simulink model "Controllo_Simulazione"  (R2020b)
settings: Solver=FixedStepDiscrete  StartTime=0.0  StopTime=5  FixedStep=0.001  RelTol=1e-3
undefined symbols (not defined in the file or in its folder): DiscIntNeverNeededParam
libraries: simulink x7, simulink_extras x2
settings Model: Creator=daniele_ravasio  LastModifiedBy=simoc

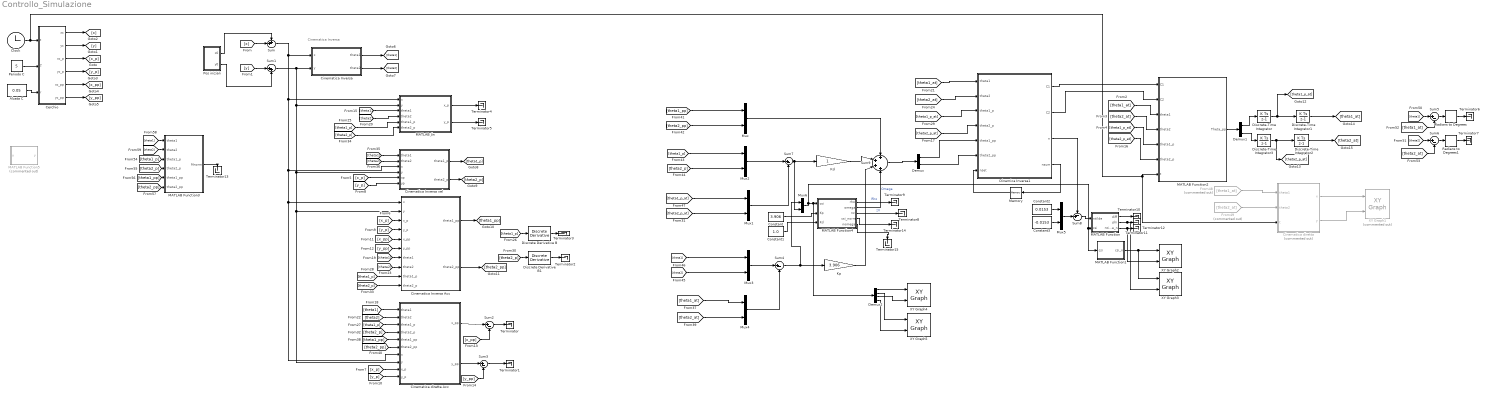
== system Controllo_Simulazione ==
  note: Cinematica Inversa
  Alzata C : Constant  Value=0.05
  Cerchio : MATLAB Function  TreatAsAtomicUnit=on
  Cinematica Inversa : MATLAB Function  TreatAsAtomicUnit=on
  Cinematica Inversa Acc : MATLAB Function  TreatAsAtomicUnit=on
  Cinematica Inversa vel : MATLAB Function  TreatAsAtomicUnit=on
  Cinematica diretta : MATLAB Function  Commented=on  TreatAsAtomicUnit=on
  Cinematica diretta Acc : MATLAB Function  TreatAsAtomicUnit=on
  Clock : Clock
  Constant : Constant  Value=3.906
  Constant1 : Constant  Value=1.0
  Constant2 : Constant  Value=0.0153
  Constant3 : Constant  Value=-0.0153
  Demux : Demux  Outputs=2
  Demux1 : Demux  Outputs=2
  Demux2 : Demux
  Dinamica Inversa1 : MATLAB Function  TreatAsAtomicUnit=on
  Discrete Derivative B : simulink/Discrete/Discrete Derivative  gainval=1.0  ICPrevScaledInput=0.0  OutMin=[]  OutMax=[]  OutDataType=fixdt(1, 16)  OutScaling=2^-10  DoSatur=off
  Discrete Derivative B1 : simulink/Discrete/Discrete Derivative  gainval=1.0  ICPrevScaledInput=0.0  OutMin=[]  OutMax=[]  OutDataType=fixdt(1, 16)  OutScaling=2^-10  DoSatur=off
  Discrete-Time Integrator : DiscreteIntegrator  SampleTime=-1  ICPrevOutput=DiscIntNeverNeededParam  ICPrevScaledInput=DiscIntNeverNeededParam
  Discrete-Time Integrator1 : DiscreteIntegrator  InitialCondition=deg2rad(100)  SampleTime=-1  ICPrevOutput=DiscIntNeverNeededParam  ICPrevScaledInput=DiscIntNeverNeededParam
  Discrete-Time Integrator2 : DiscreteIntegrator  InitialCondition=deg2rad(80)  SampleTime=-1  ICPrevOutput=DiscIntNeverNeededParam  ICPrevScaledInput=DiscIntNeverNeededParam
  Discrete-Time Integrator3 : DiscreteIntegrator  SampleTime=-1  ICPrevOutput=DiscIntNeverNeededParam  ICPrevScaledInput=DiscIntNeverNeededParam
  From48 : From  Commented=on  GotoTag=theta1_at
  From49 : From  Commented=on  GotoTag=theta2_at
  Kd : Gain
  Kp : Gain  Gain=3.906
  MATLAB Function : MATLAB Function  TreatAsAtomicUnit=on
  MATLAB Function1 : MATLAB Function  TreatAsAtomicUnit=on
  MATLAB Function2 : MATLAB Function  TreatAsAtomicUnit=on
  MATLAB Function3 : MATLAB Function  TreatAsAtomicUnit=on
  MATLAB Function4 : MATLAB Function  TreatAsAtomicUnit=on
  MATLAB Function5 : MATLAB Function  Commented=on  TreatAsAtomicUnit=on
  MATLAB Jin : MATLAB Function  TreatAsAtomicUnit=on
  Memory : Memory
  Mux{,1..6} (7 alike) : Mux  Inputs=2
  Periodo C : Constant  Value=5
  Pos iniziali : Subsystem
  Radians to Degrees : simulink_extras/Transformations/Radians to Degrees
  Radians to Degrees1 : simulink_extras/Transformations/Radians to Degrees
  Sum : Sum  Inputs=++|
  Sum1 : Sum  Inputs=|++
  Sum{2..7} (6 alike) : Sum  Inputs=|+-
  Sum8 : Sum  Inputs=-+|
  Sum9 : Sum  Inputs=+|+|+|+
  Terminator{,1..15} (16 alike) : Terminator
  XY Graph1 : simulink/Sinks/XY Graph  Commented=on  xmin=-0.15  xmax=0.15  ymin=0  ymax=0.5  st=0.001
  XY Graph2 : simulink/Sinks/XY Graph  xmin=0  xmax=0.01  ymin=0  ymax=0.05  st=0.001
  XY Graph3 : simulink/Sinks/XY Graph  xmin=0  xmax=0.01  ymin=0  ymax=0.1  st=0.001
  XY Graph4 : simulink/Sinks/XY Graph  xmin=0  xmax=0.01  ymin=0  ymax=0.1  st=0.001
  XY Graph5 : simulink/Sinks/XY Graph  xmin=0  xmax=0.01  ymin=0  ymax=0.1  st=0.001
  wires:
  Clock/1 -> MATLAB Function2/7(t), Cinematica diretta/3(t), Cerchio/1(t)
  Alzata C/1 -> Cerchio/3(r)
  Periodo C/1 -> Cerchio/2(T)
  Mux1/1 -> Sum7/2
  [x_pp] -> Sum2/2
  Cerchio/5(xc_pp) -> [x_pp]
  Pos iniziali/1(x0) -> Sum/1
  [theta1] -> Cinematica Inversa Acc/7(theta1)
  Demux/2 -> Dinamica Inversa1/6(theta2_pp)
  [theta1] -> Cinematica Inversa vel/1(theta1)
  [theta1_p] -> Discrete Derivative B/1
  [x_p] -> Cinematica Inversa vel/5(xp)
  Cinematica diretta Acc/2(y_pp) -> Sum3/1
  Cerchio/1(xc) -> [x]
  Cerchio/3(xc_p) -> [x_p]
  [theta2] -> Cinematica Inversa Acc/8(theta2)
  [theta1] -> Cinematica diretta Acc/1(theta1)
  Cinematica Inversa Acc/1(theta1_pp) -> [theta1_pp]
  Kd/1 -> Sum9/2
  Mux/1 -> Sum9/1
  Cinematica Inversa/1(theta1) -> [theta1]
  [theta2_p] -> MATLAB Jin/6(theta2_p)
  Cinematica diretta/2(y) -> XY Graph1/2
  [x_p] -> Cinematica diretta Acc/9(x_p)
  Cinematica diretta/1(x) -> XY Graph1/1
  Kp/1 -> Sum9/3
  Demux/1 -> Dinamica Inversa1/5(theta1_pp)
  Mux3/1 -> Sum4/1
  Cinematica Inversa vel/2(theta2_p) -> [theta2_p]
  Sum4/1 -> Mux6/1, Kp/1
  Mux4/1 -> Sum4/2
  [theta2] -> Cinematica Inversa vel/2(theta2)
  [theta1_p] -> Cinematica diretta Acc/3(theta1_p)
  [theta2_p] -> Cinematica diretta Acc/4(theta2_p)
  Sum3/1 -> Terminator1/1
  Mux2/1 -> Sum7/1
  MATLAB Jin/1(x_p) -> Terminator4/1
  [x] -> Sum/2
  Sum7/1 -> Mux6/2, Kd/1
  Sum9/1 -> Demux/1
  [y_pp] -> Cinematica Inversa Acc/6(y_pp)
  Pos iniziali/2(y0) -> Sum1/2
  [theta1_p] -> MATLAB Jin/5(theta1_p)
  [theta1_pp] -> Cinematica diretta Acc/5(theta1_pp)
  [y] -> Sum1/1
  Cinematica Inversa vel/1(theta1_p) -> [theta1_p]
  [y_p] -> Cinematica Inversa vel/6(yp)
  [y_pp] -> Sum3/2
  [theta1] -> MATLAB Jin/3(theta1)
  [y_p] -> Cinematica Inversa Acc/4(y_p)
  Cinematica Inversa/2(theta2) -> [theta2]
  Sum2/1 -> Terminator/1
  [theta2] -> MATLAB Jin/4(theta2)
  [x_p] -> Cinematica Inversa Acc/3(x_p)
  [y_p] -> Cinematica diretta Acc/10(y_p)
  [x_pp] -> Cinematica Inversa Acc/5(x_pp)
  [theta2] -> Cinematica diretta Acc/2(theta2)
  MATLAB Jin/2(y_p) -> Terminator5/1
  [theta2_p] -> Cinematica Inversa Acc/10(theta2_p)
  Cinematica diretta Acc/1(x_pp) -> Sum2/1
  [theta2_p] -> Discrete Derivative B1/1
  Cerchio/4(yc_p) -> [y_p]
  Cerchio/6(yc_pp) -> [y_pp]
  [theta1_p] -> Cinematica Inversa Acc/9(theta1_p)
  [theta2_pp] -> Cinematica diretta Acc/6(theta2_pp)
  Cerchio/2(yc) -> [y]
  Sum1/1 -> Cinematica Inversa Acc/2(y), Cinematica diretta Acc/8(y), Cinematica Inversa vel/4(y), MATLAB Jin/2(y), Cinematica Inversa/2(y)
  Sum/1 -> Cinematica Inversa Acc/1(x), Cinematica diretta Acc/7(x), Cinematica Inversa vel/3(x), MATLAB Jin/1(x), Cinematica Inversa/1(x)
  [theta1_pp] -> Mux/1
  [theta2_pp] -> Mux/2
  [theta2_p] -> Mux2/2
  [theta1_p] -> Mux2/1
  Dinamica Inversa1/1(C1) -> MATLAB Function2/1(C1)
  Dinamica Inversa1/2(C2) -> MATLAB Function2/2(C2)
  MATLAB Function2/1(Theta_pp) -> Demux1/1
  Demux1/1 -> Discrete-Time Integrator/1
  Demux1/2 -> Discrete-Time Integrator3/1
  Discrete-Time Integrator3/1 -> Discrete-Time Integrator2/1, [theta2_p_at]
  Discrete-Time Integrator/1 -> Discrete-Time Integrator1/1, [theta1_p_at]
  [theta1_at] -> MATLAB Function2/3(theta1)
  [theta2_at] -> MATLAB Function2/4(theta2)
  Discrete-Time Integrator1/1 -> [theta1_at]
  Discrete-Time Integrator2/1 -> [theta2_at]
  [theta1_p_at] -> MATLAB Function2/5(theta1_p)
  [theta2_p_at] -> MATLAB Function2/6(theta2_p)
  [theta1_p_at] -> Dinamica Inversa1/3(theta1_p)
  [theta2_p_at] -> Dinamica Inversa1/4(theta2_p)
  [theta1_at] -> Mux4/1
  [theta2_at] -> Mux4/2
  From49/1 -> Cinematica diretta/2(theta2)
  From48/1 -> Cinematica diretta/1(theta1)
  [theta1_p_at] -> Mux1/1
  [theta2_p_at] -> Mux1/2
  [theta1] -> Mux3/1
  [theta2] -> Mux3/2
  [theta1_at] -> Dinamica Inversa1/1(theta1)
  [theta2_at] -> Dinamica Inversa1/2(theta2)
  [theta1] -> Sum5/1
  [theta1_at] -> Sum5/2
  [theta2] -> Sum6/1
  [theta2_at] -> Sum6/2
  Sum5/1 -> Radians to Degrees/1
  Radians to Degrees/1 -> Terminator6/1
  Sum6/1 -> Radians to Degrees1/1
  Radians to Degrees1/1 -> Terminator7/1
  Cinematica Inversa Acc/2(theta2_pp) -> [theta2_pp]
  Discrete Derivative B1/1 -> Terminator2/1
  Discrete Derivative B/1 -> Terminator3/1
  MATLAB Function4/2(omega) -> Sum9/4  "Omega"
  Constant/1 -> MATLAB Function4/2(Kp)
  Constant1/1 -> MATLAB Function4/3(Kd)
  MATLAB Function4/1(rho) -> Terminator9/1  "Rho"
  Dinamica Inversa1/4(nsum) -> Memory/1
  Memory/1 -> Dinamica Inversa1/7(nset)
  Dinamica Inversa1/3(n) -> Sum8/1
  Constant2/1 -> Mux5/1
  Constant3/1 -> Mux5/2
  Mux5/1 -> Sum8/2
  Sum8/1 -> MATLAB Function/1(ntilde)
  Mux6/1 -> Demux2/1, MATLAB Function4/1(csi), MATLAB Function1/1(csi), MATLAB Function/2(csi)
  MATLAB Function/1(diff) -> Terminator10/1
  MATLAB Function/2(phi) -> XY Graph3/2, Terminator11/1
  MATLAB Function1/1(csi_n) -> XY Graph3/1, XY Graph2/1
  MATLAB Function/3(ntilde_n) -> XY Graph2/2, Terminator12/1
  [theta1_p] -> MATLAB Function3/3(theta1_p)
  [theta2_p] -> MATLAB Function3/4(theta2_p)
  [theta1_pp] -> MATLAB Function3/5(theta1_pp)
  [theta2_pp] -> MATLAB Function3/6(theta2_pp)
  [theta1] -> MATLAB Function3/1(theta1)
  [theta2] -> MATLAB Function3/2(theta2)
  MATLAB Function3/1(Mnorm) -> Terminator13/1
  MATLAB Function4/4(csi_norm) -> Terminator14/1
  MATLAB Function4/5(nomega) -> Terminator15/1
  MATLAB Function4/3(nz) -> Terminator8/1  "zV"
  Demux2/1 -> XY Graph4/1
  Demux2/3 -> XY Graph4/2
  Demux2/2 -> XY Graph5/1
  Demux2/4 -> XY Graph5/2

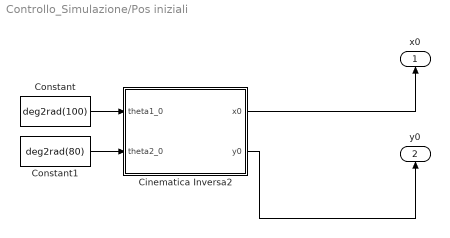
== system Controllo_Simulazione/Pos iniziali ==
  Cinematica Inversa2 : MATLAB Function  TreatAsAtomicUnit=on
  Constant : Constant  Value=deg2rad(100)
  Constant1 : Constant  Value=deg2rad(80)
  x0 : Outport
  y0 : Outport  Port=2
  wires:
  Cinematica Inversa2/1(x0) -> x0/1
  Cinematica Inversa2/2(y0) -> y0/1
  Constant/1 -> Cinematica Inversa2/1(theta1_0)
  Constant1/1 -> Cinematica Inversa2/2(theta2_0)

== matlab function Controllo_Simulazione/Cinematica diretta ==
  data: x output; theta1 input; y output; theta2 input; t input
function [x, y] = fcn(theta1, theta2,t)
d = 0.09;
l = 0.25;


A = l^2*(sin(theta2)-sin(theta1))^2 + (-2*d -l*(cos(theta2)-cos(theta1)))^2;
B = -2*l^2*d*(sin(theta2)-sin(theta1))*(cos(theta2)+cos(theta1)) + ...
    l*(sin(theta2)-sin(theta1))*(-2*d -l*(cos(theta2)-cos(theta1)))*(-2*d -2*l*cos(theta2)) - ...
    2*l*sin(theta2)*(-2*d -l*(cos(theta2)-cos(theta1)))^2;
C = l^2*d^2*(cos(theta2)+cos(theta1))^2 -l*d*(cos(theta2)+cos(theta1))*(-2*d -l*(cos(theta2)-cos(theta1)))*(-2*d -2*l*cos(theta2)) + ...
    (d^2 + 2*d*l*cos(theta2))*(-2*d - l*(cos(theta2)-cos(theta1)))^2;

% Posizione Y end-effector
y =  (-B + sqrt(B^2 - 4*A*C))/(2*A);
% Posizione X end-effector
x =  (y*l*(sin(theta2)-sin(theta1)) - l*d*(cos(theta2)+cos(theta1)))/(-2*d -l*(cos(theta2)-cos(theta1)));
end

== matlab function Controllo_Simulazione/Pos iniziali/Cinematica Inversa2 ==
  data: theta1_0 input; theta2_0 input; x0 output; y0 output
function [x0, y0] = fcn(theta1_0, theta2_0)

d = 0.09; 
l = 0.25;

A = l^2*(sin(theta2_0)-sin(theta1_0))^2 + (-2*d -l*(cos(theta2_0)-cos(theta1_0)))^2;
B = -2*l^2*d*(sin(theta2_0)-sin(theta1_0))*(cos(theta2_0)+cos(theta1_0)) + ...
    l*(sin(theta2_0)-sin(theta1_0))*(-2*d -l*(cos(theta2_0)-cos(theta1_0)))*(-2*d -2*l*cos(theta2_0)) - ...
    2*l*sin(theta2_0)*(-2*d -l*(cos(theta2_0)-cos(theta1_0)))^2;
C = l^2*d^2*(cos(theta2_0)+cos(theta1_0))^2 -l*d*(cos(theta2_0)+cos(theta1_0))*(-2*d -l*(cos(theta2_0)-cos(theta1_0)))*(-2*d -2*l*cos(theta2_0)) + ...
    (d^2 + 2*d*l*cos(theta2_0))*(-2*d - l*(cos(theta2_0)-cos(theta1_0)))^2;

% Posizione Y end-effector
y0 = (-B + sqrt(B^2 - 4*A*C))/(2*A);
% Posizione X end-effector
x0 = (y0*l*(sin(theta2_0)-sin(theta1_0)) - l*d*(cos(theta2_0)+cos(theta1_0)))/(-2*d -l*(cos(theta2_0)-cos(theta1_0)));

== matlab function Controllo_Simulazione/Cinematica Inversa ==
  data: x input; theta1 output; y input; theta2 output
function [theta1, theta2] = fcn(x, y)

d = 0.09; 
l = 0.25;

p = 2*d*l + 2*x*l;
e = 2*y*l;
f = x^2 + d^2 + y^2 + 2*x*d;
a = -2*d*l + 2*x*l;
b = +2*y*l;
c = x^2 + d^2 + y^2 - 2*x*d;



   theta1 = 2*atan2(e + sqrt(p^2 + e^2 -f^2), p +f);


   theta2 = 2*atan2(b - sqrt(a^2 + b^2 -c^2), a +c);
   if (theta2) < -deg2rad(200)
       theta2 = theta2 + 2*pi;
   end

== matlab function Controllo_Simulazione/Cinematica Inversa vel ==
  data: theta1 input; theta2 input; x input; y input; xp input; theta1_p output; yp input; theta2_p output
function [theta1_p, theta2_p] = fcn(theta1, theta2,x, y, xp, yp)

d = 0.09; 
l = 0.25;

N21 = -l*sin(theta1)*(x+d-l*cos(theta1)) + l*cos(theta1)*(y-l*sin(theta1));

N22 = -l*cos(theta2)*(y-l*sin(theta2))*(x+d-l*cos(theta1))/(x-d-l*cos(theta2)) + l*sin(theta2)*(x+d-l*cos(theta1));

D2 = y-l*sin(theta1) - (y-l*sin(theta2))*(x+d-l*cos(theta1))/(x-d-l*cos(theta2));

J21 = N21/D2;

J22 = N22/D2;

J11 = -(y-l*sin(theta2))/(x-d-l*cos(theta2))*(J21);

J12 = -(y-l*sin(theta2))/(x-d-l*cos(theta2))*(J22) -l*sin(theta2) + (y-l*sin(theta2))/(x-d-l*cos(theta2))*(l*cos(theta2));

J = [J11 J12; J21 J22];

theta_p = J^-1 * [xp; yp];
theta1_p = theta_p(1);
theta2_p = theta_p(2);

== matlab function Controllo_Simulazione/MATLAB Jin ==
  data: x input; y input; theta1 input; x_p output; theta2 input; theta1_p input; theta2_p input; y_p output
function [x_p, y_p] = fcn(x, y, theta1, theta2, theta1_p, theta2_p)

d = 0.09; 
l = 0.25;

N21 = -l*sin(theta1)*(x+d-l*cos(theta1)) + l*cos(theta1)*(y-l*sin(theta1));

N22 = -l*cos(theta2)*(y-l*sin(theta2))*(x+d-l*cos(theta1))/(x-d-l*cos(theta2)) + l*sin(theta2)*(x+d-l*cos(theta1));

D2 = y-l*sin(theta1) - (y-l*sin(theta2))*(x+d-l*cos(theta1))/(x-d-l*cos(theta2));

J21 = N21/D2;

J22 = N22/D2;

J11 = -(y-l*sin(theta2))/(x-d-l*cos(theta2))*(J21);

J12 = -(y-l*sin(theta2))/(x-d-l*cos(theta2))*(J22) -l*sin(theta2) + (y-l*sin(theta2))/(x-d-l*cos(theta2))*(l*cos(theta2));

x_p = J11*theta1_p + J12*theta2_p;
y_p = J21*theta1_p + J22*theta2_p;

== matlab function Controllo_Simulazione/Cerchio ==
  data: xc output; t input; yc output; T input; r input; xc_p output; yc_p output; xc_pp output; yc_pp output
function [xc, yc, xc_p, yc_p, xc_pp, yc_pp] = fcn(t, T, r)
xv = 0.4;
xj = 0.1;
x = t/T;
Ca = 1/((1-xv)*(xv-xj));
if ( x >= 0 && x < xj)            %acc crescente positiva
    f = Ca/xj*x;
    F = (1/2)*Ca/xj*x^2;
    G = (1/6)*Ca/xj*x^3;
    J = Ca/xj;

  elseif (x >= xj && x < (xv-xj))   %acc costante positiva
    f = Ca;
    F = Ca*x - (1/2)*Ca*xj;
    G = (1/2)*Ca*x^2 - (1/2)*Ca*xj*x + (1/6)*Ca*xj^2;
    J = 0;

  elseif( x>= (xv-xj) && x < xv)    %acc decrescente positiva
    f = -Ca/xj*x + Ca*xv/xj;
    F = -(1/2)*Ca/xj*x^2 + Ca/xj*xv*x - Ca*(xj + (1/2)/xj*xv^2 - xv);
    G = -(1/6)*Ca/xj*x^3 + (1/2)*Ca/xj*xv*x^2 - Ca*(xj + (1/2)/xj*xv^2 - xv)*x ...
        - (1/2)*Ca*xv^2  + (1/6)*Ca/xj*xv^3 + (1/2)*Ca*xv*xj;
    J = -Ca/xj;

  elseif( x>= xv && x < (1-xv))     %acc costante nulla
    f = 0;
    F = Ca*(xv - xj);
    G = Ca*(xv - xj)*x - (1/2)*Ca*xv^2 + (1/2)*Ca*xv*xj;
    J = 0;
    
  elseif( x>= (1-xv) && x < (1-xv+xj))   %acc decrescente negativa
    f = -Ca/xj*x + Ca/xj*(1-xv);
    F = -(1/2)*Ca/xj*x^2 + Ca/xj*(1-xv)*x + Ca*(xv-xj) - (1/2)*Ca/xj*(1-xv)^2;
    G = -(1/6)*Ca/xj*x^3 + (1/2)*Ca/xj*(1-xv)*x^2 + Ca*(xv-xj)*x - (1/2)*Ca/xj*(1-xv)^2*x ...
        - (1/2)*Ca*xv^2 + (1/2)*Ca*xv*xj + (1/6)*Ca/xj*(1-xv)^3;
    J = -Ca/xj;
    
  elseif( x>= (1-xv+xj) && x < (1-xj))   %acc costante negativa
    f = -Ca; 
    F = -Ca*x + Ca - (1/2)*Ca*xj;
    G = -(1/2)*Ca*x^2 + Ca*x - (1/2)*Ca*xj*x + 1 - Ca*(-(1/2)*xj + (1/6)*xj^2 + (1/2));
    J = 0;
    
  elseif( x>= (1-xj) && x <= 1)          %acc crescente negativa
    f = Ca/xj*(x-1);
    F = (1/2)*Ca/xj*x^2 - Ca/xj*x +(1/2)*Ca/xj;
    G = (1/6)*Ca/xj*x^3 - (1/2)*Ca/xj*x^2 +(1/2)*Ca/xj*x + 1 - (1/6)*Ca/xj;
    J = Ca/xj;
    
  else                                   %acc costante nulla
    f = 0;
    F = 0;
    G = 1;
    J = 0;
end
  
 alfa = G*2*pi;
 alfa_p = F*2*pi/T;
 alfa_pp = f*2*pi/(T^2);
 xc = r*cos(pi/2-alfa);
 yc = r*sin(pi/2-alfa) - r;
 xc_p = r*sin(pi/2-alfa)*alfa_p;
 yc_p = -r*cos(pi/2-alfa)*alfa_p;
 xc_pp = -r*cos(pi/2-alfa)*alfa_p^2 + r*sin(pi/2-alfa)*alfa_pp;
 yc_pp = -r*sin(pi/2-alfa)*alfa_p^2- r*cos(pi/2-alfa)*alfa_pp;

== matlab function Controllo_Simulazione/Cinematica Inversa Acc ==
  data: x input; y input; x_p input; y_p input; x_pp input; y_pp input; theta1 input; theta2 input; theta1_pp output; theta1_p input; theta2_p input; theta2_pp output
function [theta1_pp, theta2_pp] = CinInvAcc(x, y, x_p, y_p, x_pp, y_pp, theta1, theta2, theta1_p,theta2_p)

d = 0.09; 
l = 0.25;

N21 = -l*sin(theta1)*(x+d-l*cos(theta1)) + l*cos(theta1)*(y-l*sin(theta1));

N22 = -l*cos(theta2)*(y-l*sin(theta2))*(x+d-l*cos(theta1))/(x-d-l*cos(theta2)) + l*sin(theta2)*(x+d-l*cos(theta1));

D2 = y-l*sin(theta1) - (y-l*sin(theta2))*(x+d-l*cos(theta1))/(x-d-l*cos(theta2));

J21 = N21/D2;

J22 = N22/D2;

J11 = -(y-l*sin(theta2))/(x-d-l*cos(theta2))*(J21);

J12 = -(y-l*sin(theta2))/(x-d-l*cos(theta2))*(J22) -l*sin(theta2) + (y-l*sin(theta2))/(x-d-l*cos(theta2))*(l*cos(theta2));

J = [J11 J12; J21 J22];

J_p11 = ((l*cos(theta1)*(y - l*sin(theta1)) - l*sin(theta1)*(d + x - l*cos(theta1)))*(y_p - l*cos(theta2)*theta2_p))/((d - x + l*cos(theta2))*(y - l*sin(theta1) + ((y - l*sin(theta2))*(d + x - l*cos(theta1)))/(d - x + l*cos(theta2)))) - ((y - l*sin(theta2))*(l*sin(theta1)*(x_p + l*sin(theta1)*theta1_p) - l*cos(theta1)*(y_p - l*cos(theta1)*theta1_p) + l*sin(theta1)*(y - l*sin(theta1))*theta1_p + l*cos(theta1)*theta1_p*(d + x - l*cos(theta1))))/((d - x + l*cos(theta2))*(y - l*sin(theta1) + ((y - l*sin(theta2))*(d + x - l*cos(theta1)))/(d - x + l*cos(theta2)))) + ((x_p + l*sin(theta2)*theta2_p)*(y - l*sin(theta2))*(l*cos(theta1)*(y - l*sin(theta1)) - l*sin(theta1)*(d + x - l*cos(theta1))))/((d - x + l*cos(theta2))^2*(y - l*sin(theta1) + ((y - l*sin(theta2))*(d + x - l*cos(theta1)))/(d - x + l*cos(theta2)))) - ((y - l*sin(theta2))*(l*cos(theta1)*(y - l*sin(theta1)) - l*sin(theta1)*(d + x - l*cos(theta1)))*(y_p + ((x_p + l*sin(theta1)*theta1_p)*(y - l*sin(theta2)))/(d - x + l*cos(theta2)) + ((y_p - l*cos(theta2)*theta2_p)*(d + x - l*cos(theta1)))/(d - x + l*cos(theta2)) - l*cos(theta1)*theta1_p + ((x_p + l*sin(theta2)*theta2_p)*(y - l*sin(theta2))*(d + x - l*cos(theta1)))/(d - x + l*cos(theta2))^2))/((d - x + l*cos(theta2))*(y - l*sin(theta1) + ((y - l*sin(theta2))*(d + x - l*cos(theta1)))/(d - x + l*cos(theta2)))^2);
 
 
J_p12 = ((y - l*sin(theta2))*(l*sin(theta2)*(x_p + l*sin(theta1)*theta1_p) + l*cos(theta2)*theta2_p*(d + x - l*cos(theta1)) + (l*cos(theta2)*(x_p + l*sin(theta1)*theta1_p)*(y - l*sin(theta2)))/(d - x + l*cos(theta2)) + (l*cos(theta2)*(y_p - l*cos(theta2)*theta2_p)*(d + x - l*cos(theta1)))/(d - x + l*cos(theta2)) - (l*sin(theta2)*(y - l*sin(theta2))*theta2_p*(d + x - l*cos(theta1)))/(d - x + l*cos(theta2)) + (l*cos(theta2)*(x_p + l*sin(theta2)*theta2_p)*(y - l*sin(theta2))*(d + x - l*cos(theta1)))/(d - x + l*cos(theta2))^2))/((d - x + l*cos(theta2))*(y - l*sin(theta1) + ((y - l*sin(theta2))*(d + x - l*cos(theta1)))/(d - x + l*cos(theta2)))) - l*cos(theta2)*theta2_p - (l*cos(theta2)*(y_p - l*cos(theta2)*theta2_p))/(d - x + l*cos(theta2)) + ((l*sin(theta2)*(d + x - l*cos(theta1)) + (l*cos(theta2)*(y - l*sin(theta2))*(d + x - l*cos(theta1)))/(d - x + l*cos(theta2)))*(y_p - l*cos(theta2)*theta2_p))/((d - x + l*cos(theta2))*(y - l*sin(theta1) + ((y - l*sin(theta2))*(d + x - l*cos(theta1)))/(d - x + l*cos(theta2)))) - (l*cos(theta2)*(x_p + l*sin(theta2)*theta2_p)*(y - l*sin(theta2)))/(d - x + l*cos(theta2))^2 + ((x_p + l*sin(theta2)*theta2_p)*(l*sin(theta2)*(d + x - l*cos(theta1)) + (l*cos(theta2)*(y - l*sin(theta2))*(d + x - l*cos(theta1)))/(d - x + l*cos(theta2)))*(y - l*sin(theta2)))/((d - x + l*cos(theta2))^2*(y - l*sin(theta1) + ((y - l*sin(theta2))*(d + x - l*cos(theta1)))/(d - x + l*cos(theta2)))) - ((l*sin(theta2)*(d + x - l*cos(theta1)) + (l*cos(theta2)*(y - l*sin(theta2))*(d + x - l*cos(theta1)))/(d - x + l*cos(theta2)))*(y - l*sin(theta2))*(y_p + ((x_p + l*sin(theta1)*theta1_p)*(y - l*sin(theta2)))/(d - x + l*cos(theta2)) + ((y_p - l*cos(theta2)*theta2_p)*(d + x - l*cos(theta1)))/(d - x + l*cos(theta2)) - l*cos(theta1)*theta1_p + ((x_p + l*sin(theta2)*theta2_p)*(y - l*sin(theta2))*(d + x - l*cos(theta1)))/(d - x + l*cos(theta2))^2))/((d - x + l*cos(theta2))*(y - l*sin(theta1) + ((y - l*sin(theta2))*(d + x - l*cos(theta1)))/(d - x + l*cos(theta2)))^2) + (l*sin(theta2)*(y - l*sin(theta2))*theta2_p)/(d - x + l*cos(theta2));
 
 
J_p21 = - (l*sin(theta1)*(x_p + l*sin(theta1)*theta1_p) - l*cos(theta1)*(y_p - l*cos(theta1)*theta1_p) + l*sin(theta1)*(y - l*sin(theta1))*theta1_p + l*cos(theta1)*theta1_p*(d + x - l*cos(theta1)))/(y - l*sin(theta1) + ((y - l*sin(theta2))*(d + x - l*cos(theta1)))/(d - x + l*cos(theta2))) - ((l*cos(theta1)*(y - l*sin(theta1)) - l*sin(theta1)*(d + x - l*cos(theta1)))*(y_p + ((x_p + l*sin(theta1)*theta1_p)*(y - l*sin(theta2)))/(d - x + l*cos(theta2)) + ((y_p - l*cos(theta2)*theta2_p)*(d + x - l*cos(theta1)))/(d - x + l*cos(theta2)) - l*cos(theta1)*theta1_p + ((x_p + l*sin(theta2)*theta2_p)*(y - l*sin(theta2))*(d + x - l*cos(theta1)))/(d - x + l*cos(theta2))^2))/(y - l*sin(theta1) + ((y - l*sin(theta2))*(d + x - l*cos(theta1)))/(d - x + l*cos(theta2)))^2;
 
 
J_p22 = (l*sin(theta2)*(x_p + l*sin(theta1)*theta1_p) + l*cos(theta2)*theta2_p*(d + x - l*cos(theta1)) + (l*cos(theta2)*(x_p + l*sin(theta1)*theta1_p)*(y - l*sin(theta2)))/(d - x + l*cos(theta2)) + (l*cos(theta2)*(y_p - l*cos(theta2)*theta2_p)*(d + x - l*cos(theta1)))/(d - x + l*cos(theta2)) - (l*sin(theta2)*(y - l*sin(theta2))*theta2_p*(d + x - l*cos(theta1)))/(d - x + l*cos(theta2)) + (l*cos(theta2)*(x_p + l*sin(theta2)*theta2_p)*(y - l*sin(theta2))*(d + x - l*cos(theta1)))/(d - x + l*cos(theta2))^2)/(y - l*sin(theta1) + ((y - l*sin(theta2))*(d + x - l*cos(theta1)))/(d - x + l*cos(theta2))) - ((l*sin(theta2)*(d + x - l*cos(theta1)) + (l*cos(theta2)*(y - l*sin(theta2))*(d + x - l*cos(theta1)))/(d - x + l*cos(theta2)))*(y_p + ((x_p + l*sin(theta1)*theta1_p)*(y - l*sin(theta2)))/(d - x + l*cos(theta2)) + ((y_p - l*cos(theta2)*theta2_p)*(d + x - l*cos(theta1)))/(d - x + l*cos(theta2)) - l*cos(theta1)*theta1_p + ((x_p + l*sin(theta2)*theta2_p)*(y - l*sin(theta2))*(d + x - l*cos(theta1)))/(d - x + l*cos(theta2))^2))/(y - l*sin(theta1) + ((y - l*sin(theta2))*(d + x - l*cos(theta1)))/(d - x + l*cos(theta2)))^2;
 

J_p = [J_p11, J_p12
    J_p21, J_p22];
     
Theta_pp = (inv(J))*([x_pp; y_pp] - J_p*[theta1_p; theta2_p]);

theta1_pp = Theta_pp(1,1);
theta2_pp = Theta_pp(2,1);

== matlab function Controllo_Simulazione/Cinematica diretta Acc ==
  data: theta1 input; x_pp output; theta2 input; theta1_p input; theta2_p input; theta1_pp input; theta2_pp input; x input; y input; x_p input; y_p input; y_pp output
function [x_pp, y_pp] = fcn(theta1, theta2, theta1_p, theta2_p, theta1_pp, theta2_pp, x, y, x_p, y_p)

d = 0.09; 
l = 0.25;

A = x_p^2 + 2*l*sin(theta2)*x_p*theta2_p + (l*sin(theta2)*theta2_p)^2 + (x-d-l*cos(theta2))*(l*cos(theta2)*theta2_p^2 + l*sin(theta2)*theta2_pp) +...
    y_p^2 - 2*l*cos(theta2)*y_p*theta2_p + (l*cos(theta2)*theta2_p)^2 + (y-l*sin(theta2))*(l*sin(theta2)*theta2_p^2 - l*cos(theta2)*theta2_pp);

B = x_p^2 + 2*l*sin(theta1)*x_p*theta1_p + (l*sin(theta1)*theta1_p)^2 + (x+d-l*cos(theta1))*(l*cos(theta1)*theta1_p^2 + l*sin(theta1)*theta1_pp) +...
    y_p^2 - 2*l*cos(theta1)*y_p*theta1_p + (l*cos(theta1)*theta1_p)^2 + (y-l*sin(theta1))*(l*sin(theta1)*theta1_p^2 - l*cos(theta1)*theta1_pp);

y_pp = (B*(x-d-l*cos(theta2))/(x+d-l*cos(theta1)) - A)/(y-l*sin(theta2) - (x-d-l*cos(theta2))/(x+d-l*cos(theta1))*(y-l*sin(theta1)));

x_pp = (-y_pp*(y-l*sin(theta1)) - B)/(x+d-l*cos(theta1));

== matlab function Controllo_Simulazione/Dinamica Inversa1 ==
  data: theta1 input; C1 output; C2 output; n output; theta2 input; theta1_p input; theta2_p input; theta1_pp input; theta2_pp input; nset input; nsum output
function [C1, C2,n, nsum] = Dinamica_Inversa(theta1,theta2,theta1_p,theta2_p,theta1_pp,theta2_pp, nset)
d = 0.09;
l = 0.25;
m = 2.9;
me = 0.36;
pv = 0.02;
Jv = 6.4e-06;
J = 5.22e-02;

A1 = cos(theta1)*theta1_p^2 + sin(theta1)*theta1_pp;
A2 = cos(theta2)*theta2_p^2 + sin(theta2)*theta2_pp;
B1 = -sin(theta1)*theta1_p^2 + cos(theta1)*theta1_pp;
B2 = -sin(theta2)*theta2_p^2 + cos(theta2)*theta2_pp;

theta3 = 2*atan((sin(theta2) - sin(theta1) + ((cos(theta2) - cos(theta1) + 18/25)^2 - ((cos(theta2) - cos(theta1) + 18/25)^2/2 +...
    (sin(theta1) - sin(theta2))^2/2)^2 + (sin(theta1) - sin(theta2))^2)^(1/2))/(cos(theta2) - cos(theta1) +...
    (cos(theta2) - cos(theta1) + 18/25)^2/2 + (sin(theta1) - sin(theta2))^2/2 + 18/25));

theta4 = -2*atan((sin(theta2) - sin(theta1) + ((cos(theta2) - cos(theta1) + 18/25)^2 - ((cos(theta2) - cos(theta1) + 18/25)^2/2 + (sin(theta1) -...
    sin(theta2))^2/2)^2 + (sin(theta1) - sin(theta2))^2)^(1/2))/(cos(theta1) - cos(theta2) + (cos(theta2) - cos(theta1) + 18/25)^2/2 +...
    (sin(theta1) -sin(theta2))^2/2 - 18/25));

N13 = cos(theta4)/sin(theta4)*sin(theta1)-cos(theta1);
N23 = cos(theta2)-cos(theta4)/sin(theta4)*sin(theta2);
D13 = cos(theta3)-cos(theta4)/sin(theta4)*sin(theta3);

theta3_p = (theta1_p*(N13)+theta2_p*(N23))/D13;

N21 = sin(theta1)*(cos(theta3)/sin(theta3) - cos(theta4)/sin(theta4)) +...
    cos(theta4)/sin(theta4)*sin(theta1) - cos(theta1);
N22 = -sin(theta2)*(cos(theta3)/sin(theta3) - cos(theta4)/sin(theta4)) -...
    cos(theta4)/sin(theta4)*sin(theta2) + cos(theta2);
D2 = sin(theta4)*(cos(theta3)/sin(theta3) - cos(theta4)/sin(theta4));

theta4_p = theta1_p*(N21/D2)+ theta2_p*(N22/D2);

J34 = [N13/D13, N23/D13; N21/D2, N22/D2];

theta3_pp = (-B1 +B2 + sin(theta3)*theta3_p^2 - sin(theta4)*theta4_p^2 + cos(theta4)/sin(theta4)*(A1 - A2 + cos(theta3)*theta3_p^2 - cos(theta4)*theta4_p^2))/...
    (cos(theta3) - cos(theta4)/sin(theta4)*sin(theta3));

theta4_pp = (A1 - A2 + cos(theta3)*theta3_p^2 - cos(theta4)*theta4_p^2 + sin(theta3)*theta3_pp)/sin(theta4);

N11 = cos(theta4)/sin(theta4)*sin(theta1)-cos(theta1);
N12 = cos(theta2)-cos(theta4)/sin(theta4)*sin(theta2);
D1 = cos(theta3)-cos(theta4)/sin(theta4)*sin(theta3);

N21 = sin(theta1)*(cos(theta3)/sin(theta3) - cos(theta4)/sin(theta4)) +...
    cos(theta4)/sin(theta4)*sin(theta1) - cos(theta1);
N22 = -sin(theta2)*(cos(theta3)/sin(theta3) - cos(theta4)/sin(theta4)) -...
    cos(theta4)/sin(theta4)*sin(theta2) + cos(theta2);
D2 = sin(theta4)*(cos(theta3)/sin(theta3) - cos(theta4)/sin(theta4));

N11p =  (-1)/(sin(theta4)^2)*theta4_p*sin(theta1) + cos(theta4)/sin(theta4)*cos(theta1)*theta1_p + sin(theta1)*theta1_p;

N12p = -(-1)/(sin(theta4)^2)*theta4_p*sin(theta2) - cos(theta4)/sin(theta4)*cos(theta2)*theta2_p - sin(theta2)*theta2_p;

D1p = -sin(theta3)*theta3_p -(-1)/(sin(theta4)^2)*theta4_p*sin(theta3) - cos(theta4)/sin(theta4)*cos(theta3)*theta3_p;

N21p = cos(theta1)*theta1_p*(cos(theta3)/sin(theta3) - cos(theta4)/sin(theta4)) + sin(theta1)*((-1)/(sin(theta3)^2)*theta3_p + 1/(sin(theta4)^2)*theta4_p) + ...
    (-1)/(sin(theta4)^2)*theta4_p*sin(theta1) + cos(theta4)/sin(theta4)*cos(theta1)*theta1_p + sin(theta1)*theta1_p;

N22p = -cos(theta2)*theta2_p*(cos(theta3)/sin(theta3) - cos(theta4)/sin(theta4)) - sin(theta2)*((-1)/(sin(theta3)^2)*theta3_p + 1/(sin(theta4)^2)*theta4_p) - ...
    (-1)/(sin(theta4)^2)*theta4_p*sin(theta2) - cos(theta4)/sin(theta4)*cos(theta2)*theta2_p - sin(theta2)*theta2_p;

D2p = cos(theta4)*theta4_p*(cos(theta3)/sin(theta3) - cos(theta4)/sin(theta4)) + sin(theta4)*((-1)/(sin(theta3)^2)*theta3_p + 1/(sin(theta4)^2)*theta4_p);

J34p = [(N11p*D1 - N11*D1p)/(D1^2), (N12p*D1 - N12*D1p)/(D1^2);(N21p*D2 - N21*D2p)/(D2^2), (N22p*D2 - N22*D2p)/(D2^2)];

J1 = [-0.5*l*sin(theta1), 0;
        0.5*l*cos(theta1), 0]; 
J1p = [-0.5*l*cos(theta1)*theta1_p, 0;
       -0.5*l*sin(theta1)*theta1_p, 0];

J2 = [0, -0.5*l*sin(theta2);
       0,  0.5*l*cos(theta2)]; 
J2p = [0, -0.5*l*cos(theta2)*theta2_p;
       0, -0.5*l*sin(theta2)*theta2_p];

J3 = [ -l*(sin(theta1)+0.5*sin(theta3)*J34(1,1)), -l*(0.5*sin(theta3)*J34(1,2));
        l*(cos(theta1)+0.5*cos(theta3)*J34(1,1)),  l*(0.5*cos(theta3)*J34(1,2))];
J3p = [ -l*(cos(theta1)*theta1_p+0.5*cos(theta3)*theta3_p*J34(1,1)+0.5*sin(theta3)*J34p(1,1)), -l*(0.5*cos(theta3)*theta3_p*J34(1,2)+0.5*sin(theta3)*J34p(1,2));
        l*(-sin(theta1)*theta1_p-0.5*sin(theta3)*theta3_p*J34(1,1)+0.5*cos(theta3)*J34p(1,1)), l*(-0.5*sin(theta3)*theta3_p*J34(1,2)+0.5*cos(theta3)*J34p(1,2))];

J4 = [ -l*0.5*sin(theta4)*J34(2,1), -l*(sin(theta2)+0.5*sin(theta4)*J34(2,2));
         l*0.5*cos(theta4)*J34(2,1),  l*(cos(theta2)+0.5*cos(theta4)*J34(2,2))];
J4p = [ -l*(0.5*cos(theta4)*theta4_p*J34(2,1)+0.5*sin(theta4)*J34p(2,1)), -l*(cos(theta2)*theta2_p+0.5*cos(theta4)*theta4_p*J34(2,2)+0.5*sin(theta4)*J34p(2,2));
        l*(-0.5*sin(theta4)*theta4_p*J34(2,1)+0.5*cos(theta4)*J34p(2,1)), l*(-sin(theta2)*theta2_p-0.5*sin(theta4)*theta4_p*J34(2,2)+0.5*cos(theta4)*J34p(2,2))];

JE = [ -l*(sin(theta1)+sin(theta3)*J34(1,1)), -l*(sin(theta3)*J34(1,2));
        l*(cos(theta1)+cos(theta3)*J34(1,1)),  l*(cos(theta3)*J34(1,2))];
JEp = [ -l*(cos(theta1)*theta1_p+cos(theta3)*theta3_p*J34(1,1)+sin(theta3)*J34p(1,1)), -l*(cos(theta3)*theta3_p*J34(1,2)+sin(theta3)*J34p(1,2));
        l*(-sin(theta1)*theta1_p-sin(theta3)*theta3_p*J34(1,1)+cos(theta3)*J34p(1,1)), l*(-sin(theta3)*theta3_p*J34(1,2)+cos(theta3)*J34p(1,2))];
  
  
M = ((J+1.7e-05*64^2)*eye(2) + m*(J1')*J1 + m*(J2')*J2 + J*(J34')*J34 + m*(J3')*J3 + m*(J4')*J4 + me*(JE')*JE);
K = (m*(J1')*J1p + m*(J2')*J2p + J*(J34')*J34p + m*(J3')*J3p + m*(J4')*J4p + me*(JE')*JEp);

C = M*[theta1_pp; theta2_pp] + K*[theta1_p; theta2_p];
n = K*[theta1_p; theta2_p];
nsum = nset+n;
Jm = [1.7e-05, 0; 0, 1.7e-05];
Jtrasm = [1/64, 0; 0, 1/64];
Thetam_pp = Jtrasm^-1*[theta1_pp; theta2_pp];
Thetam_p = Jtrasm^-1*[theta1_p; theta2_p];

Cm = Jtrasm*C + Jm*Thetam_pp;
Mm = (Jtrasm'*M*Jtrasm + Jm);

Km = (Jtrasm'*K*Jtrasm);
Cm = Mm*Thetam_pp  +  Km*Thetam_p;

% Mm_ = Jm;
% DMm = Mm-Jm;
% D = DMm*Thetam_pp + Km*Thetam_p;
% Aol = [zeros(2,2) eye(2,2); zeros(2,2), zeros(2,2)];
% Bt = [zeros(2,2); Mm_^-1];
% Acl = Aol - Bt*[Kp Kd];


C1 = C(1,1);
C2 = C(2,1);

== matlab function Controllo_Simulazione/MATLAB Function1 ==
  data: csi input; csi_n output
function csi_n = fcn(csi)

csi_n = norm(csi);

== matlab function Controllo_Simulazione/MATLAB Function ==
  data: ntilde input; diff output; csi input; phi output; ntilde_n output
function [diff, phi, ntilde_n] = fcn(ntilde,csi)
a0 = 0.05;
a1 = 5;
a2 = -50; %
phi = a0 + a1*norm(csi) + a2*norm(csi)^2;
diff = norm(ntilde) - phi;
ntilde_n = norm(ntilde);

== matlab function Controllo_Simulazione/MATLAB Function2 ==
  data: C1 input; Theta_pp output; C2 input; theta1 input; theta2 input; theta1_p input; theta2_p input; t input
function Theta_pp  = fcn(C1, C2, theta1, theta2, theta1_p, theta2_p,t)

if t <= 0.001
    theta1 = deg2rad(100);
    theta1_p = 0;
    theta2 = deg2rad(80);
    theta2_p = 0;
end


d = 0.09;
l = 0.25;
m = 2.9;
me = 0.36;
pv = 0.02;
Jv = 6.4e-06;
J = 5.22e-02;


theta3 = 2*atan((sin(theta2) - sin(theta1) + ((cos(theta2) - cos(theta1) + 18/25)^2 - ((cos(theta2) - cos(theta1) + 18/25)^2/2 +...
    (sin(theta1) - sin(theta2))^2/2)^2 + (sin(theta1) - sin(theta2))^2)^(1/2))/(cos(theta2) - cos(theta1) +...
    (cos(theta2) - cos(theta1) + 18/25)^2/2 + (sin(theta1) - sin(theta2))^2/2 + 18/25));

theta4 = -2*atan((sin(theta2) - sin(theta1) + ((cos(theta2) - cos(theta1) + 18/25)^2 - ((cos(theta2) - cos(theta1) + 18/25)^2/2 + (sin(theta1) -...
    sin(theta2))^2/2)^2 + (sin(theta1) - sin(theta2))^2)^(1/2))/(cos(theta1) - cos(theta2) + (cos(theta2) - cos(theta1) + 18/25)^2/2 +...
    (sin(theta1) -sin(theta2))^2/2 - 18/25));

N13 = cos(theta4)/sin(theta4)*sin(theta1)-cos(theta1);
N23 = cos(theta2)-cos(theta4)/sin(theta4)*sin(theta2);
D13 = cos(theta3)-cos(theta4)/sin(theta4)*sin(theta3);

theta3_p = (theta1_p*(N13)+theta2_p*(N23))/D13;

N21 = sin(theta1)*(cos(theta3)/sin(theta3) - cos(theta4)/sin(theta4)) +...
    cos(theta4)/sin(theta4)*sin(theta1) - cos(theta1);
N22 = -sin(theta2)*(cos(theta3)/sin(theta3) - cos(theta4)/sin(theta4)) -...
    cos(theta4)/sin(theta4)*sin(theta2) + cos(theta2);
D2 = sin(theta4)*(cos(theta3)/sin(theta3) - cos(theta4)/sin(theta4));

theta4_p = theta1_p*(N21/D2)+ theta2_p*(N22/D2);

J34 = [N13/D13, N23/D13; N21/D2, N22/D2];

N11 = cos(theta4)/sin(theta4)*sin(theta1)-cos(theta1);
N12 = cos(theta2)-cos(theta4)/sin(theta4)*sin(theta2);
D1 = cos(theta3)-cos(theta4)/sin(theta4)*sin(theta3);

N21 = sin(theta1)*(cos(theta3)/sin(theta3) - cos(theta4)/sin(theta4)) +...
    cos(theta4)/sin(theta4)*sin(theta1) - cos(theta1);
N22 = -sin(theta2)*(cos(theta3)/sin(theta3) - cos(theta4)/sin(theta4)) -...
    cos(theta4)/sin(theta4)*sin(theta2) + cos(theta2);
D2 = sin(theta4)*(cos(theta3)/sin(theta3) - cos(theta4)/sin(theta4));

N11p =  (-1)/(sin(theta4)^2)*theta4_p*sin(theta1) + cos(theta4)/sin(theta4)*cos(theta1)*theta1_p + sin(theta1)*theta1_p;

N12p = -(-1)/(sin(theta4)^2)*theta4_p*sin(theta2) - cos(theta4)/sin(theta4)*cos(theta2)*theta2_p - sin(theta2)*theta2_p;

D1p = -sin(theta3)*theta3_p -(-1)/(sin(theta4)^2)*theta4_p*sin(theta3) - cos(theta4)/sin(theta4)*cos(theta3)*theta3_p;

N21p = cos(theta1)*theta1_p*(cos(theta3)/sin(theta3) - cos(theta4)/sin(theta4)) + sin(theta1)*((-1)/(sin(theta3)^2)*theta3_p + 1/(sin(theta4)^2)*theta4_p) + ...
    (-1)/(sin(theta4)^2)*theta4_p*sin(theta1) + cos(theta4)/sin(theta4)*cos(theta1)*theta1_p + sin(theta1)*theta1_p;

N22p = -cos(theta2)*theta2_p*(cos(theta3)/sin(theta3) - cos(theta4)/sin(theta4)) - sin(theta2)*((-1)/(sin(theta3)^2)*theta3_p + 1/(sin(theta4)^2)*theta4_p) - ...
    (-1)/(sin(theta4)^2)*theta4_p*sin(theta2) - cos(theta4)/sin(theta4)*cos(theta2)*theta2_p - sin(theta2)*theta2_p;

D2p = cos(theta4)*theta4_p*(cos(theta3)/sin(theta3) - cos(theta4)/sin(theta4)) + sin(theta4)*((-1)/(sin(theta3)^2)*theta3_p + 1/(sin(theta4)^2)*theta4_p);

J34p = [(N11p*D1 - N11*D1p)/(D1^2), (N12p*D1 - N12*D1p)/(D1^2);(N21p*D2 - N21*D2p)/(D2^2), (N22p*D2 - N22*D2p)/(D2^2)];

J1 = [-0.5*l*sin(theta1), 0;
        0.5*l*cos(theta1), 0]; 
J1p = [-0.5*l*cos(theta1)*theta1_p, 0;
       -0.5*l*sin(theta1)*theta1_p, 0];

J2 = [0, -0.5*l*sin(theta2);
       0,  0.5*l*cos(theta2)]; 
J2p = [0, -0.5*l*cos(theta2)*theta2_p;
       0, -0.5*l*sin(theta2)*theta2_p];

J3 = [ -l*(sin(theta1)+0.5*sin(theta3)*J34(1,1)), -l*(0.5*sin(theta3)*J34(1,2));
        l*(cos(theta1)+0.5*cos(theta3)*J34(1,1)),  l*(0.5*cos(theta3)*J34(1,2))];
J3p = [ -l*(cos(theta1)*theta1_p+0.5*cos(theta3)*theta3_p*J34(1,1)+0.5*sin(theta3)*J34p(1,1)), -l*(0.5*cos(theta3)*theta3_p*J34(1,2)+0.5*sin(theta3)*J34p(1,2));
        l*(-sin(theta1)*theta1_p-0.5*sin(theta3)*theta3_p*J34(1,1)+0.5*cos(theta3)*J34p(1,1)), l*(-0.5*sin(theta3)*theta3_p*J34(1,2)+0.5*cos(theta3)*J34p(1,2))];

J4 = [ -l*0.5*sin(theta4)*J34(2,1), -l*(sin(theta2)+0.5*sin(theta4)*J34(2,2));
         l*0.5*cos(theta4)*J34(2,1),  l*(cos(theta2)+0.5*cos(theta4)*J34(2,2))];
J4p = [ -l*(0.5*cos(theta4)*theta4_p*J34(2,1)+0.5*sin(theta4)*J34p(2,1)), -l*(cos(theta2)*theta2_p+0.5*cos(theta4)*theta4_p*J34(2,2)+0.5*sin(theta4)*J34p(2,2));
        l*(-0.5*sin(theta4)*theta4_p*J34(2,1)+0.5*cos(theta4)*J34p(2,1)), l*(-sin(theta2)*theta2_p-0.5*sin(theta4)*theta4_p*J34(2,2)+0.5*cos(theta4)*J34p(2,2))];

JE = [ -l*(sin(theta1)+sin(theta3)*J34(1,1)), -l*(sin(theta3)*J34(1,2));
        l*(cos(theta1)+cos(theta3)*J34(1,1)),  l*(cos(theta3)*J34(1,2))];
JEp = [ -l*(cos(theta1)*theta1_p+cos(theta3)*theta3_p*J34(1,1)+sin(theta3)*J34p(1,1)), -l*(cos(theta3)*theta3_p*J34(1,2)+sin(theta3)*J34p(1,2));
        l*(-sin(theta1)*theta1_p-sin(theta3)*theta3_p*J34(1,1)+cos(theta3)*J34p(1,1)), l*(-sin(theta3)*theta3_p*J34(1,2)+cos(theta3)*J34p(1,2))];
  
  
M = (J*eye(2) + m*(J1')*J1 + m*(J2')*J2 + J*(J34')*J34 + m*(J3')*J3 + m*(J4')*J4 + me*(JE')*JE);
K = (m*(J1')*J1p + m*(J2')*J2p + J*(J34')*J34p + m*(J3')*J3p + m*(J4')*J4p + me*(JE')*JEp);
Jm = [1.7e-05, 0; 0, 1.7e-05];
Jtrasm = [1/64, 0; 0, 1/64];
Mm = (Jtrasm'*M*Jtrasm + Jm);
Km = (Jtrasm'*K*Jtrasm);
Thetam_p = 64*[theta1_p;theta2_p];
Theta_pp = M^-1*(-Km*[theta1_p; theta2_p]+[C1; C2]);

== matlab function Controllo_Simulazione/MATLAB Function3 ==
  data: theta1 input; Mnorm output; theta2 input; theta1_p input; theta2_p input; theta1_pp input; theta2_pp input
function Mnorm  = fcn(theta1,theta2,theta1_p,theta2_p,theta1_pp,theta2_pp)

d = 0.09;
l = 0.25;
m = 2.9;
me = 0.36;
pv = 0.02;
Jv = 6.4e-06;
J = 5.22e-02;

 
A1 = cos(theta1)*theta1_p^2 + sin(theta1)*theta1_pp;
A2 = cos(theta2)*theta2_p^2 + sin(theta2)*theta2_pp;
B1 = -sin(theta1)*theta1_p^2 + cos(theta1)*theta1_pp;
B2 = -sin(theta2)*theta2_p^2 + cos(theta2)*theta2_pp;


theta3 = 2*atan((sin(theta2) - sin(theta1) + ((cos(theta2) - cos(theta1) + 18/25)^2 - ((cos(theta2) - cos(theta1) + 18/25)^2/2 +...
    (sin(theta1) - sin(theta2))^2/2)^2 + (sin(theta1) - sin(theta2))^2)^(1/2))/(cos(theta2) - cos(theta1) +...
    (cos(theta2) - cos(theta1) + 18/25)^2/2 + (sin(theta1) - sin(theta2))^2/2 + 18/25));

theta4 = -2*atan((sin(theta2) - sin(theta1) + ((cos(theta2) - cos(theta1) + 18/25)^2 - ((cos(theta2) - cos(theta1) + 18/25)^2/2 + (sin(theta1) -...
    sin(theta2))^2/2)^2 + (sin(theta1) - sin(theta2))^2)^(1/2))/(cos(theta1) - cos(theta2) + (cos(theta2) - cos(theta1) + 18/25)^2/2 +...
    (sin(theta1) -sin(theta2))^2/2 - 18/25));

N13 = cos(theta4)/sin(theta4)*sin(theta1)-cos(theta1);
N23 = cos(theta2)-cos(theta4)/sin(theta4)*sin(theta2);
D13 = cos(theta3)-cos(theta4)/sin(theta4)*sin(theta3);

theta3_p = (theta1_p*(N13)+theta2_p*(N23))/D13;

N21 = sin(theta1)*(cos(theta3)/sin(theta3) - cos(theta4)/sin(theta4)) +...
    cos(theta4)/sin(theta4)*sin(theta1) - cos(theta1);
N22 = -sin(theta2)*(cos(theta3)/sin(theta3) - cos(theta4)/sin(theta4)) -...
    cos(theta4)/sin(theta4)*sin(theta2) + cos(theta2);
D2 = sin(theta4)*(cos(theta3)/sin(theta3) - cos(theta4)/sin(theta4));

theta4_p = theta1_p*(N21/D2)+ theta2_p*(N22/D2);

J34 = [N13/D13, N23/D13; N21/D2, N22/D2];

theta3_pp = (-B1 +B2 + sin(theta3)*theta3_p^2 - sin(theta4)*theta4_p^2 + cos(theta4)/sin(theta4)*(A1 - A2 + cos(theta3)*theta3_p^2 - cos(theta4)*theta4_p^2))/...
    (cos(theta3) - cos(theta4)/sin(theta4)*sin(theta3));

theta4_pp = (A1 - A2 + cos(theta3)*theta3_p^2 - cos(theta4)*theta4_p^2 + sin(theta3)*theta3_pp)/sin(theta4);

N11 = cos(theta4)/sin(theta4)*sin(theta1)-cos(theta1);
N12 = cos(theta2)-cos(theta4)/sin(theta4)*sin(theta2);
D1 = cos(theta3)-cos(theta4)/sin(theta4)*sin(theta3);

N21 = sin(theta1)*(cos(theta3)/sin(theta3) - cos(theta4)/sin(theta4)) +...
    cos(theta4)/sin(theta4)*sin(theta1) - cos(theta1);
N22 = -sin(theta2)*(cos(theta3)/sin(theta3) - cos(theta4)/sin(theta4)) -...
    cos(theta4)/sin(theta4)*sin(theta2) + cos(theta2);
D2 = sin(theta4)*(cos(theta3)/sin(theta3) - cos(theta4)/sin(theta4));

N11p =  (-1)/(sin(theta4)^2)*theta4_p*sin(theta1) + cos(theta4)/sin(theta4)*cos(theta1)*theta1_p + sin(theta1)*theta1_p;

N12p = -(-1)/(sin(theta4)^2)*theta4_p*sin(theta2) - cos(theta4)/sin(theta4)*cos(theta2)*theta2_p - sin(theta2)*theta2_p;

D1p = -sin(theta3)*theta3_p -(-1)/(sin(theta4)^2)*theta4_p*sin(theta3) - cos(theta4)/sin(theta4)*cos(theta3)*theta3_p;

N21p = cos(theta1)*theta1_p*(cos(theta3)/sin(theta3) - cos(theta4)/sin(theta4)) + sin(theta1)*((-1)/(sin(theta3)^2)*theta3_p + 1/(sin(theta4)^2)*theta4_p) + ...
    (-1)/(sin(theta4)^2)*theta4_p*sin(theta1) + cos(theta4)/sin(theta4)*cos(theta1)*theta1_p + sin(theta1)*theta1_p;

N22p = -cos(theta2)*theta2_p*(cos(theta3)/sin(theta3) - cos(theta4)/sin(theta4)) - sin(theta2)*((-1)/(sin(theta3)^2)*theta3_p + 1/(sin(theta4)^2)*theta4_p) - ...
    (-1)/(sin(theta4)^2)*theta4_p*sin(theta2) - cos(theta4)/sin(theta4)*cos(theta2)*theta2_p - sin(theta2)*theta2_p;

D2p = cos(theta4)*theta4_p*(cos(theta3)/sin(theta3) - cos(theta4)/sin(theta4)) + sin(theta4)*((-1)/(sin(theta3)^2)*theta3_p + 1/(sin(theta4)^2)*theta4_p);

J34p = [(N11p*D1 - N11*D1p)/(D1^2), (N12p*D1 - N12*D1p)/(D1^2);(N21p*D2 - N21*D2p)/(D2^2), (N22p*D2 - N22*D2p)/(D2^2)];

J1 = [-0.5*l*sin(theta1), 0;
        0.5*l*cos(theta1), 0]; 
J1p = [-0.5*l*cos(theta1)*theta1_p, 0;
       -0.5*l*sin(theta1)*theta1_p, 0];

J2 = [0, -0.5*l*sin(theta2);
       0,  0.5*l*cos(theta2)]; 
J2p = [0, -0.5*l*cos(theta2)*theta2_p;
       0, -0.5*l*sin(theta2)*theta2_p];

J3 = [ -l*(sin(theta1)+0.5*sin(theta3)*J34(1,1)), -l*(0.5*sin(theta3)*J34(1,2));
        l*(cos(theta1)+0.5*cos(theta3)*J34(1,1)),  l*(0.5*cos(theta3)*J34(1,2))];
J3p = [ -l*(cos(theta1)*theta1_p+0.5*cos(theta3)*theta3_p*J34(1,1)+0.5*sin(theta3)*J34p(1,1)), -l*(0.5*cos(theta3)*theta3_p*J34(1,2)+0.5*sin(theta3)*J34p(1,2));
        l*(-sin(theta1)*theta1_p-0.5*sin(theta3)*theta3_p*J34(1,1)+0.5*cos(theta3)*J34p(1,1)), l*(-0.5*sin(theta3)*theta3_p*J34(1,2)+0.5*cos(theta3)*J34p(1,2))];

J4 = [ -l*0.5*sin(theta4)*J34(2,1), -l*(sin(theta2)+0.5*sin(theta4)*J34(2,2));
         l*0.5*cos(theta4)*J34(2,1),  l*(cos(theta2)+0.5*cos(theta4)*J34(2,2))];
J4p = [ -l*(0.5*cos(theta4)*theta4_p*J34(2,1)+0.5*sin(theta4)*J34p(2,1)), -l*(cos(theta2)*theta2_p+0.5*cos(theta4)*theta4_p*J34(2,2)+0.5*sin(theta4)*J34p(2,2));
        l*(-0.5*sin(theta4)*theta4_p*J34(2,1)+0.5*cos(theta4)*J34p(2,1)), l*(-sin(theta2)*theta2_p-0.5*sin(theta4)*theta4_p*J34(2,2)+0.5*cos(theta4)*J34p(2,2))];

JE = [ -l*(sin(theta1)+sin(theta3)*J34(1,1)), -l*(sin(theta3)*J34(1,2));
        l*(cos(theta1)+cos(theta3)*J34(1,1)),  l*(cos(theta3)*J34(1,2))];
JEp = [ -l*(cos(theta1)*theta1_p+cos(theta3)*theta3_p*J34(1,1)+sin(theta3)*J34p(1,1)), -l*(cos(theta3)*theta3_p*J34(1,2)+sin(theta3)*J34p(1,2));
        l*(-sin(theta1)*theta1_p-sin(theta3)*theta3_p*J34(1,1)+cos(theta3)*J34p(1,1)), l*(-sin(theta3)*theta3_p*J34(1,2)+cos(theta3)*J34p(1,2))];
  
  
M = ((J+1.7e-05*64^2)*eye(2) + m*(J1')*J1 + m*(J2')*J2 + J*(J34')*J34 + m*(J3')*J3 + m*(J4')*J4 + me*(JE')*JE);
K = (m*(J1')*J1p + m*(J2')*J2p + J*(J34')*J34p + m*(J3')*J3p + m*(J4')*J4p + me*(JE')*JEp);
Mnorm = norm(M);
end

== matlab function Controllo_Simulazione/MATLAB Function5 ==
  data: u input; y output
function y = fcn(u)
x = t/T;

if( x >= 0 && x <= 1 )
    J = 60-180*3*x+360*(x^2);
    f = 60*x-180*(x^2)+120*(x^3);
    F = 30*(x^2)-60*(x^3)+30*(x^4);
    G = 10*(x^3)-15*(x^4)+6*(x^5);
else
    J=0;
    f=0;
    F=0;
    G=0;
end

== matlab function Controllo_Simulazione/MATLAB Function4 ==
  data: rho output; csi input; omega output; nz output; Kp input; Kd input; csi_norm output; nomega output
function [rho,omega,nz,csi_norm,nomega ] = fcn(csi,Kp,Kd)
% Mm e Nm si riescono a ricavare dallo script TestMatriciTheta

Maxnorm =  0.609; %3.3415; %1.4604e+04;
Minnorm =  0.420; %0.0012; %9.5631e+03;
alpha = (Maxnorm-Minnorm)/(Maxnorm+Minnorm);
Mhat = 2/(Maxnorm+Minnorm)*eye(2);

% Calcolo Phi(||Csi||)
alpha0 = 0.05;
alpha1 = 5;
alpha2 = -5;

csiH = csi;
y = norm(csiH);
phi = alpha0+alpha1*y+alpha2*y.^2;
%% Calcolo H,P,Q
% P ? definita positiva
P = eye(4);

Ht = [0,0,-Kp,0; 
    0,0,0,-Kp;
    1,0,-Kd,0;
    0,1,0,-Kd];
H = Ht';

Q = [ (Kd^2 + Kp^2 + Kp)/(2*Kd*Kp),0 1/(2*Kp),0;
    0, (Kd^2 + Kp^2 + Kp)/(2*Kd*Kp),0, 1/(2*Kp); 
    1/(2*Kp),0, (Kp + 1)/(2*Kd*Kp),0;
    0,1/(2*Kp),0,(Kp + 1)/(2*Kd*Kp)];
%% Calcolo D e z, zV
D = [zeros(2);eye(2)];
z = D'*Q*csiH; % Il risultato ? una 2x1 [2x4][4x4][4x1]
epsilon = 0.00025;
if norm(z) < epsilon
    zV = z/epsilon;
else
    zV = z/norm(z);
end
Qm = 1.1;
% norma di omega = rho
K = [Kp,0,Kd,0; 0,Kp,0,Kd];
%y = theta_pp + K*csiH+omega;
%eta = (eye(2)-M^-1*Mhat)*y-M^-1*ntilde;

Bm = Maxnorm;
b0 = (alpha*Qm+alpha0*Bm)/(1-alpha); %[1]+[1][2,2] ERR
b1 = (alpha*norm(K)+alpha1*Bm)/(1-alpha); %[1]+[2,4][2,2] ERR
b2 = (alpha2*Bm)/(1-alpha); %[1]+[1][2,2] ERR
%rho = (1/(1-alpha))*(alpha*Qm+alpha*norm(K)*norm(CsiH)+Mm*phi);
% rho = b0+b1*norm(csiH)+b2*norm(csiH)^2;
rho = 0.28;
csi_norm = norm(csiH);
omega = rho*zV;
nomega = norm(omega);
nz = norm(z);
